simulink model "Verification_des_performences_du_correcteur"  (R2017a)
settings: Solver=VariableStepAuto  StartTime=0.0  StopTime=10.0  RelTol=1e-3
values from neighbouring files (symbols this model uses):
  Den = [1 1 1]    [LeScript.m]    (also in LesDonnées.mat)
  Num = [1 1]    [LeScript.m]    (also in LesDonnées.mat)
settings Model: Creator=PC  LastModifiedBy=PC

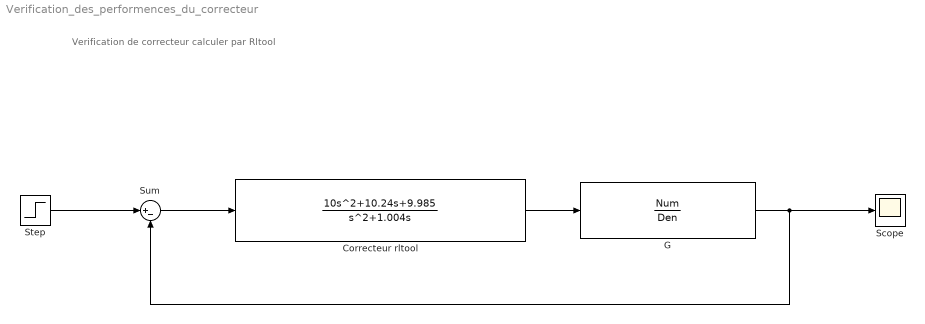
== system Verification_des_performences_du_correcteur ==
  note: Verification de correcteur calculer par Rltool
  " G" : TransferFcn  Numerator=Num  Denominator=Den
  "Correcteur rltool " : TransferFcn  Numerator=[10 10.24 9.985]  Denominator=[1 1.004 0]
  Scope : Scope
  Step : Step  Time=0  SampleTime=0
  Sum : Sum  Inputs=|+-
  wires:
  Step/1 -> Sum/1
  Sum/1 -> "Correcteur rltool "/1
  " G"/1 -> Sum/2, Scope/1
  "Correcteur rltool "/1 -> " G"/1
